simulink model "sensor_capacitive_transduction_manual"  (R2022a)
settings: Solver=VariableStepAuto  StartTime=0.0  StopTime=20  RelTol=1e-3
values from neighbouring files (symbols this model uses):
  k = 1.2    [run_frequency_sweep.m]
  r = 0.2    [run_frequency_sweep.m]
  x0 = 0    [measure_frequency_point.m]
  y0 = 0    [measure_frequency_point.m]
undefined symbols (not defined in the file or in its folder): alpha_x, d, epsA, G_C, noise_seed, noise_Ts, noise_variance, q_adc, S_C, tau_amp, V_adc_max, V_adc_min, V_max, V_min, V_offset, V_offset_est
settings Model: Creator=HJL  LastModifiedBy=HJL

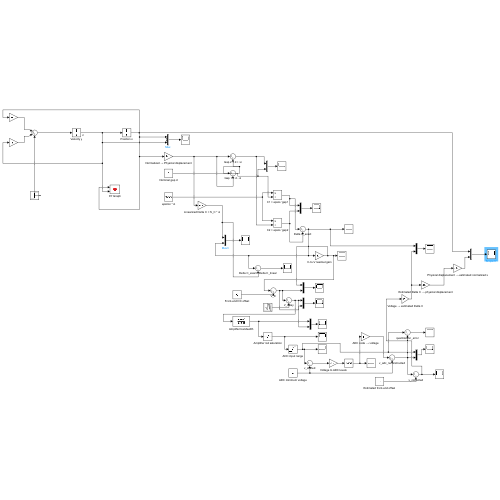
[thumbnail: Simulink's stored preview of the top-level diagram]
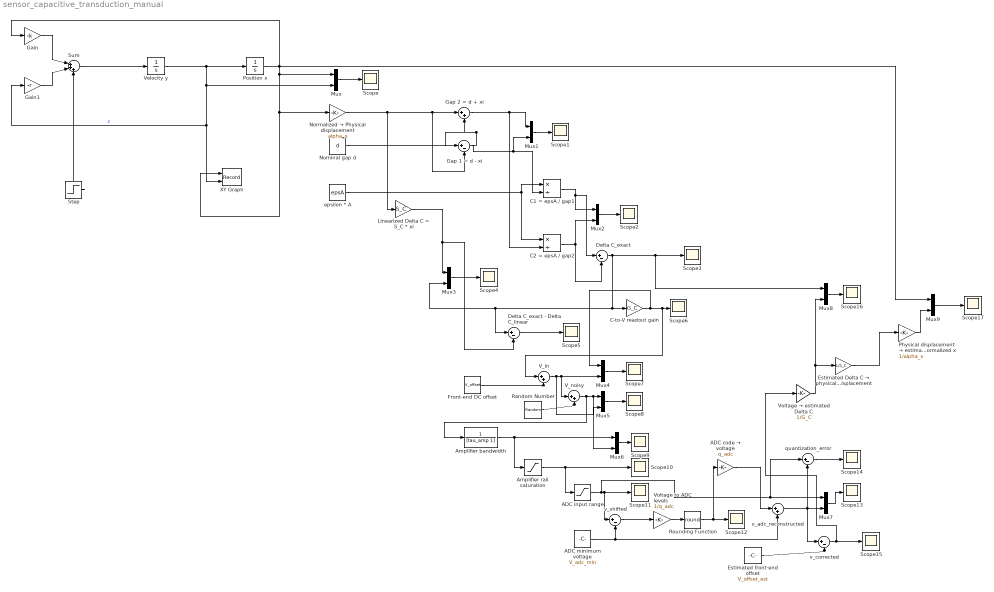
== system sensor_capacitive_transduction_manual ==
  ADC code → voltage : Gain  Gain=q_adc
  ADC input range : Saturate  UpperLimit=V_adc_max  LowerLimit=V_adc_min
  ADC minimum voltage : Constant  Value=V_adc_min
  Amplifier bandwidth : TransferFcn  Denominator=[tau_amp 1]
  Amplifier rail saturation : Saturate  UpperLimit=V_max  LowerLimit=V_min
  C-to-V readout gain : Gain  Gain=G_C
  C1 = epsA / gap1 : Product  Inputs=*/
  C2 = epsA / gap2 : Product  Inputs=*/
  Delta C_exact : Sum  Inputs=|+-
  Delta C_exact - Delta C_linear : Sum  Inputs=|+-
  Estimated Delta C → physical displacement : Gain  Gain=1/S_C
  Estimated front-end offset : Constant  Value=V_offset_est
  Front-end DC offset : Constant  Value=V_offset
  Gain : Gain  Gain=-k
  Gain1 : Gain  Gain=-r
  Gap 1 = d - xi : Sum  Inputs=|+-
  Gap 2 = d + xi : Sum  Inputs=|++
  Linearized Delta C = S_C * xi : Gain  Gain=S_C
  Mux : Mux  Inputs=3
  Mux{1..9} (9 alike) : Mux  Inputs=2
  Nominal gap d : Constant  Value=d
  Normalized → Physical displacement : Gain  Gain=alpha_x
  Physical displacement → estimated normalized x : Gain  Gain=1/alpha_x
  Position x : Integrator  InitialCondition=x0
  Random Number : RandomNumber  Variance=noise_variance  Seed=noise_seed  SampleTime=noise_Ts
  Rounding Function : Rounding  Operator=round
  Scope{,1..17} (18 alike) : Scope
  Step : Step  SampleTime=0
  Sum : Sum  Inputs=|+++
  V_in : Sum  Inputs=|++
  V_noisy : Sum  Inputs=|++
  Velocity y : Integrator  InitialCondition=y0
  Voltage to ADC levels : Gain  Gain=1/q_adc
  Voltage → estimated Delta C : Gain  Gain=1/G_C
  XY Graph : Record  FileSettingsInternal="{\"entries\":[{\"content\":{\"excelSettings\":{\"content\":{},\"type\":\"Streamout.ExcelSettings\"}},\"type\":\"Streamout.FileSettingStorage\",\"uuid\":\"91bc3ad7-c5af-44e6-9390-bc02b2f654e3\"}],\"packageUris\":[\"http://schema.mathworks.com/mf0/streamout_blocks/R2020a\"],\"version\":\"1.0\"}"  Layout=[1 1]  SignalsInternal="{\"entries\":[{\"content\":{\"signals\":[{\"content\":{\"blockPath\":[\"sensor_capacitive_transduction_manual/XY Graph\"],\"channel\":[],\"dimensions\":[1],\"domain\":\"sensor_capacitive_transduction_manual/XY Graph\",\"lineColor\":\"#fe330a\",\"plots\":[1],\"port\":1,\"sid\":[\"\"],\"signalID\":2587,\"signalName\":\"Position x\"},\"type\":\"RecordBlkView.Signal\",\"uuid\":\"65d63ea1-cab3-4728-b428-ce542938dc43\"},{\"content\":{\"blockPath\":[\"sensor_capacitive_transduction_manual/XY Graph\"],\"channel\":[],\"dimensions\":[1],\"domain\":\"sensor_capacitive_transduction_manual/XY Graph\",\"lineColor\":\"#22b573\",\"plots\":[1],\"port\":2,\"sid\":[\"\"],\"signalID\":2591,\"signalName\":\"2\"},\"type\":\"RecordBlkView.Signal\",\"uuid\":\"14ce9288-a101-4af7-a7fa-d453474b8600\"}]},\"type\":\"RecordBlkView.InputSignals\",\"uuid\":\"dd60b7db-3615-4923-a2ae-6e6d615683af\"}],\"packageUris\":[\"http://schema.mathworks.com/mf0/streamout_blocks/R2020a\"],\"version\":\"1.0\"}"  VisualizationBindings="{\"xyplotplugin\":{\"info\":[{\"series\":[{\"bindingParametersList\":[{\"parameter\":\"X-Axis\",\"signalID\":2587,\"signalName\":\"Position x\"},{\"parameter\":\"Y-Axis\",\"signalID\":2591,\"signalName\":\"2\"}],\"seriesID\":6115}],\"subplotID\":1}]}}"  CompatibilityTag=XY
  epsilon * A : Constant  Value=epsA
  quantization_error : Sum  Inputs=|+-
  v_adc_reconstructed : Sum  Inputs=|++
  v_corrected : Sum  Inputs=|+-
  v_shifted : Sum  Inputs=|+-
  wires:
  Gain1/1 -> Sum/2
  Gain/1 -> Sum/1
  Sum/1 -> Velocity y/1
  Position x/1 -> Mux9/1, Gain/1, Normalized → Physical displacement/1, XY Graph/1, Mux/1
  Velocity y/1 -> XY Graph/2, Gain1/1, Mux/3, Position x/1  "2"
  Step/1 -> Sum/3
  Mux/1 -> Scope/1
  Nominal gap d/1 -> Gap 1 = d - xi/1, Gap 2 = d + xi/2
  Normalized → Physical displacement/1 -> Linearized Delta C = S_C * xi/1, Gap 2 = d + xi/1, Gap 1 = d - xi/2
  Gap 2 = d + xi/1 -> Mux1/1, C2 = epsA / gap2/2
  Gap 1 = d - xi/1 -> C1 = epsA / gap1/2, Mux1/2
  Mux1/1 -> Scope1/1
  epsilon * A/1 -> C2 = epsA / gap2/1, C1 = epsA / gap1/1
  Mux2/1 -> Scope2/1
  C1 = epsA / gap1/1 -> Delta C_exact/1, Mux2/1
  C2 = epsA / gap2/1 -> Delta C_exact/2, Mux2/2
  Delta C_exact/1 -> C-to-V readout gain/1, Delta C_exact - Delta C_linear/1, Mux3/2, Mux8/1, Scope3/1
  Linearized Delta C = S_C * xi/1 -> Delta C_exact - Delta C_linear/2, Mux3/1
  Mux3/1 -> Scope4/1
  Delta C_exact - Delta C_linear/1 -> Scope5/1
  C-to-V readout gain/1 -> Mux4/1, V_in/1, Scope6/1
  Front-end DC offset/1 -> V_in/2
  V_in/1 -> Mux5/2, V_noisy/1, Mux4/2
  Mux4/1 -> Scope7/1
  Random Number/1 -> V_noisy/2
  V_noisy/1 -> Mux6/2, Mux5/1, Amplifier bandwidth/1
  Mux5/1 -> Scope8/1
  Amplifier bandwidth/1 -> Amplifier rail saturation/1, Mux6/1
  Mux6/1 -> Scope9/1
  Amplifier rail saturation/1 -> Scope10/1, ADC input range/1
  ADC input range/1 -> quantization_error/1, Mux7/1, v_shifted/1, Scope11/1
  ADC minimum voltage/1 -> v_adc_reconstructed/2, v_shifted/2
  v_shifted/1 -> Voltage to ADC levels/1
  Voltage to ADC levels/1 -> Rounding Function/1
  Rounding Function/1 -> ADC code → voltage/1, Scope12/1
  ADC code → voltage/1 -> v_adc_reconstructed/1
  v_adc_reconstructed/1 -> Mux7/2, v_corrected/1, quantization_error/2
  Mux7/1 -> Scope13/1
  quantization_error/1 -> Scope14/1
  Estimated front-end offset/1 -> v_corrected/2
  v_corrected/1 -> Voltage → estimated Delta C/1, Scope15/1
  Voltage → estimated Delta C/1 -> Estimated Delta C → physical displacement/1, Mux8/2
  Mux8/1 -> Scope16/1
  Estimated Delta C → physical displacement/1 -> Physical displacement → estimated normalized x/1
  Physical displacement → estimated normalized x/1 -> Mux9/2
  Mux9/1 -> Scope17/1
